simulink model "q_heli_2d_open_loop"  (Simulink 7.7)
settings: Solver=ode1  StartTime=0.0  StopTime=inf  FixedStep=0.002  RelTol=1e-3
values from neighbouring files (symbols this model uses):
  JOYSTICK_X_DZ = 0.25    [setup_lab_heli_2d.m]
  JOYSTICK_Y_DZ = 0.25    [setup_lab_heli_2d.m]
  K_AMP = 3    [setup_lab_heli_2d.m]
  K_EC_P = - 2 * pi / ( 4 * 1024 )    (= -0.00153398078789)    [setup_lab_heli_2d.m]
  K_EC_Y = 2 * pi / ( 8 * 1024 )    (= 0.000766990393943)    [setup_lab_heli_2d.m]
  K_JOYSTICK_V_X = 10    [setup_lab_heli_2d.m]
  K_JOYSTICK_V_Y = 5    [setup_lab_heli_2d.m]
  theta_0 = -40.5*pi/180    (= -0.706858347058)    [setup_lab_heli_2d.m]
  VMAX_AMP_P = 24    [setup_lab_heli_2d.m]
  VMAX_AMP_Y = 15    [setup_lab_heli_2d.m]
  wcf = 2 * pi * 20    (= 125.663706144)    [setup_lab_heli_2d.m]
  zetaf = 0.85    [setup_lab_heli_2d.m]
undefined symbols (not defined in the file or in its folder): HIL, qc_get_step_size
libraries: quarc_library x4, simulink_extras x3
settings Model: Creator=MLevis  LastModifiedBy=pmartin  SimulationMode=external  ExtModeTrigDuration=50000  BufferReuse=off
settings SolverCC: PositivePriorityOrder=on
settings OptimizationCC: BooleanDataType=off  InlineInvariantSignals=on  OptimizeBlockIOStorage=off  BufferReuse=off  ExpressionFolding=off  LocalBlockOutputs=off  InitFltsAndDblsToZero=on
settings DebuggingCC: SaveWithParameterizedLinksMsg=none  SignalResolutionControl=TryResolveAllWithWarning  MultiTaskDSMMsg=warning  MultiTaskCondExecSysMsg=none  StrictBusMsg=None
settings RTWCC: SystemTargetFile=quarc_windows.tlc  TemplateMakefile=quarc_default_tmf  Description=QuaRC Win32 Target  ProcessScript=quarc_windows_make_rtw_hook  IncludeERTFirstTime=on
settings STFCustomTargetCC: TargetFcnLib=ansi_tfl_tmw.mat  TargetPreCompLibLocation=C:\PROGRA~3\QUARC\lib\2012b\windows\release  GeneratePreprocessorConditionals=Disable all  SystemTargetFile=quarc_windows.tlc
settings GRTTargetCC: TargetFcnLib=ansi_tfl_tmw.mat  TargetPreCompLibLocation=C:\PROGRA~3\QUARC\lib\2012b\windows\release  ParMdlRefBuildCompliant=off  CompOptLevelCompliant=off  MatFileLogging=off  ExtMode=on  ExtModeMexFile=quarc_comm

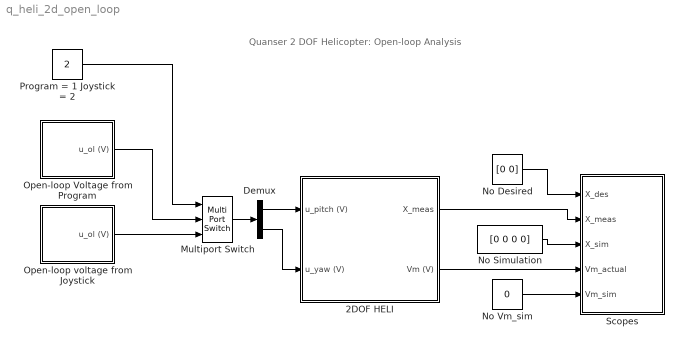
== system q_heli_2d_open_loop ==
  note: Quanser 2 DOF Helicopter:
      | Open-loop Analysis
  2DOF HELI : Subsystem
  Demux : Demux  Outputs=2
  Multiport Switch : MultiPortSwitch  Inputs=2
  No Desired : Constant  Value=[0 0]
  No Simulation : Constant  Value=[0 0 0 0]
  No Vm_sim : Constant  Value=0
  Open-loop Voltage from Program : Subsystem
  Open-loop voltage from Joystick : Subsystem
  Program = 1 Joystick = 2 : Constant  Value=2
  Scopes : Subsystem
  wires:
  Open-loop Voltage from Program/1(u_ol (V)) -> Multiport Switch/2
  Program = 1 Joystick = 2/1 -> Multiport Switch/1
  Open-loop voltage from Joystick/1(u_ol (V)) -> Multiport Switch/3
  Multiport Switch/1 -> Demux/1
  Demux/1 -> 2DOF HELI/1(u_pitch (V))
  Demux/2 -> 2DOF HELI/2(u_yaw (V))
  2DOF HELI/1(X_meas) -> Scopes/2(X_meas)
  2DOF HELI/2(Vm (V)) -> Scopes/4(Vm_actual)
  No Desired/1 -> Scopes/1(X_des)
  No Simulation/1 -> Scopes/3(X_sim)
  No Vm_sim/1 -> Scopes/5(Vm_sim)

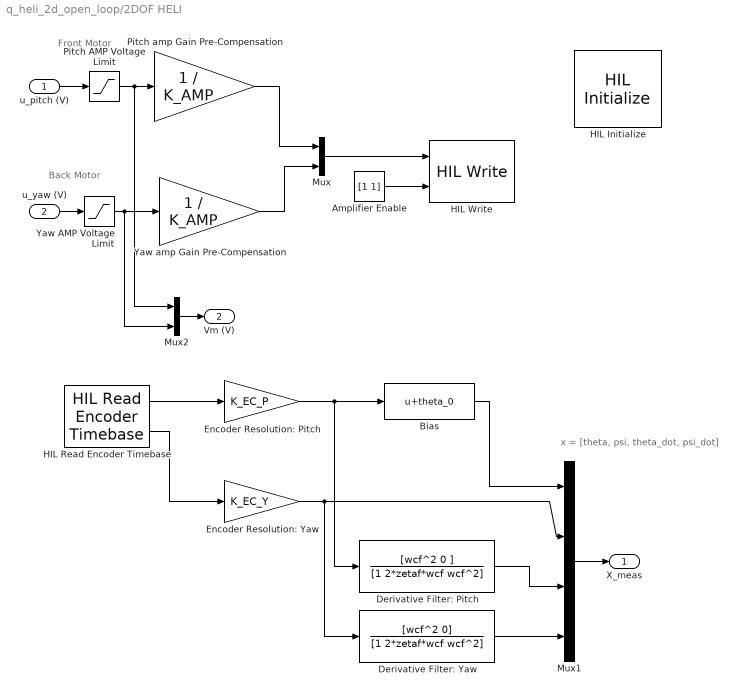
== system q_heli_2d_open_loop/2DOF HELI ==
  note: Back Motor
  note: Front Motor
  note: x = [theta, psi, theta_dot, psi_dot]
  u_pitch (V) : Inport
  u_yaw (V) : Inport  Port=2
  Amplifier Enable : Constant  Value=[1 1]
  Bias : Bias  Bias=theta_0
  Derivative Filter: Pitch : TransferFcn  Numerator=[wcf^2 0 ]  Denominator=[1 2*zetaf*wcf wcf^2]
  Derivative Filter: Yaw : TransferFcn  Numerator=[wcf^2 0]  Denominator=[1 2*zetaf*wcf wcf^2]
  "Encoder Resolution: Pitch " : Gain  Gain=K_EC_P
  Encoder Resolution: Yaw : Gain  Gain=K_EC_Y
  HIL Initialize : quarc_library/Data Acquisition/Generic/Configuration/HIL Initialize  object_name=HIL-1  board_type=q2_usb  board_number=0  board_options=d0=digital;d1=digital;led=auto;update_rate=normal;decimation=1  exclusive=off  active=on  hardware_clocks=[0]  clock_modes=[]  initial_clock_frequencies=[]  set_clock_params_at_start=off  set_clock_params_at_switch_in=off  set_clock_frequencies_at_start=off  set_clock_frequencies_at_switch_in=off  analog_input_channels=[0:1]  analog_input_maximums=10  analog_input_minimums=-10  set_analog_input_params_at_start=on  set_analog_input_params_at_switch_in=off  analog_output_channels=[0:1]  analog_output_maximums=10  analog_output_minimums=-10  initial_analog_outputs=[0]  final_analog_outputs=[0]  watchdog_analog_outputs=0  set_analog_output_params_at_start=on  set_analog_output_params_at_switch_in=off  set_analog_outputs_at_start=on  set_analog_outputs_at_switch_in=off  set_analog_outputs_at_terminate=on  set_analog_outputs_at_switch_out=off  set_analog_outputs_on_watchdog=off  digital_input_channels=[]  digital_output_channels=[0:1]  digital_output_configuration=[]  initial_digital_outputs=[0]  final_digital_outputs=[0]  watchdog_digital_outputs=[0]  set_digital_output_params_at_start=off  set_digital_output_params_at_switch_in=off  set_digital_outputs_at_start=on  set_digital_outputs_at_switch_in=off  set_digital_outputs_at_terminate=on  set_digital_outputs_at_switch_out=off  set_digital_outputs_on_watchdog=on  encoder_channels=[0:1]  quadrature=[4]  encoder_filter_frequency=[]  initial_encoder_counts=[0]  set_encoder_params_at_start=on  set_encoder_params_at_switch_in=off  set_encoder_counts_at_start=on  set_encoder_counts_at_switch_in=off  pwm_channels=[]  pwm_modes=[0]  pwm_frequency=1/0.020  pwm_configuration=[]  pwm_alignment=[]  pwm_polarity=[]  pwm_leading_deadband=[]  pwm_trailing_deadband=[]  initial_pwm_outputs=[0]  final_pwm_outputs=[0]  watchdog_pwm_outputs=[0]  set_pwm_params_at_start=on  set_pwm_params_at_switch_in=off  set_pwm_outputs_at_start=on  set_pwm_outputs_at_switch_in=off  set_pwm_outputs_at_terminate=on  set_pwm_outputs_at_switch_out=off  set_pwm_outputs_on_watchdog=off  other_output_channels=[]  initial_other_outputs=[]  final_other_outputs=[]  watchdog_other_outputs=[]  set_other_outputs_at_start=off  set_other_outputs_at_switch_in=off  set_other_outputs_at_terminate=off  set_other_outputs_at_switch_out=off  set_other_outputs_on_watchdog=off
  HIL Read Encoder Timebase : quarc_library/Data Acquisition/Generic/Timebases/HIL Read Encoder Timebase  object_name=HIL-1  clock=0  channels=[0:1]  samples_in_buffer=max(ceil(1/qc_get_step_size), 1)  active=on  vector_output=off  data_type_mode=Inherit via back propagation  data_type=double
  HIL Write : quarc_library/Data Acquisition/Generic/Immediate I//O/HIL Write  object_name=HIL-1  analog_channels=[0:1]  pwm_channels=[]  digital_channels=[0:1]  other_channels=[]  sample_time=-1  active=off  vector_input=on
  Mux : Mux  Inputs=2
  Mux1 : Mux
  Mux2 : Mux  Inputs=2
  Pitch AMP Voltage Limit : Saturate  UpperLimit=VMAX_AMP_P  LowerLimit=- VMAX_AMP_P
  Pitch amp Gain Pre-Compensation : Gain  Gain=1 / K_AMP  SaturateOnIntegerOverflow=on  OutDataTypeStr=Inherit: Same as input  ParamDataTypeStr=Inherit: Same as input
  Yaw AMP Voltage Limit : Saturate  UpperLimit=VMAX_AMP_Y  LowerLimit=- VMAX_AMP_Y
  Yaw amp Gain Pre-Compensation : Gain  Gain=1 / K_AMP  SaturateOnIntegerOverflow=on  OutDataTypeStr=Inherit: Same as input  ParamDataTypeStr=Inherit: Same as input
  X_meas : Outport
  Vm (V) : Outport  Port=2
  wires:
  Amplifier Enable/1 -> HIL Write/2
  Encoder Resolution: Yaw/1 -> Mux1/2, Derivative Filter: Yaw/1
  Mux2/1 -> Vm (V)/1
  Yaw amp Gain Pre-Compensation/1 -> Mux/2
  Pitch amp Gain Pre-Compensation/1 -> Mux/1
  Mux1/1 -> X_meas/1
  u_yaw (V)/1 -> Yaw AMP Voltage Limit/1
  u_pitch (V)/1 -> Pitch AMP Voltage Limit/1
  Yaw AMP Voltage Limit/1 -> Mux2/2, Yaw amp Gain Pre-Compensation/1
  Pitch AMP Voltage Limit/1 -> Mux2/1, Pitch amp Gain Pre-Compensation/1
  Mux/1 -> HIL Write/1
  HIL Read Encoder Timebase/1 -> "Encoder Resolution: Pitch "/1
  "Encoder Resolution: Pitch "/1 -> Bias/1, Derivative Filter: Pitch/1
  HIL Read Encoder Timebase/2 -> Encoder Resolution: Yaw/1
  Bias/1 -> Mux1/1
  Derivative Filter: Pitch/1 -> Mux1/3
  Derivative Filter: Yaw/1 -> Mux1/4

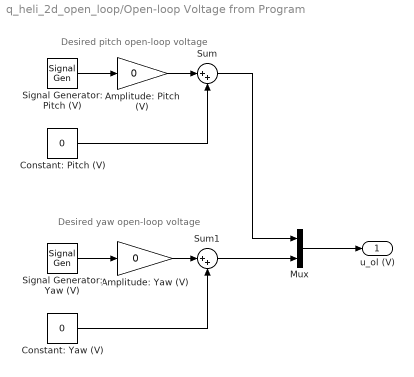
== system q_heli_2d_open_loop/Open-loop Voltage from Program ==
  note: Desired yaw open-loop voltage
  note: Desired pitch open-loop voltage
  Amplitude: Pitch (V) : Gain  Gain=0
  Amplitude: Yaw (V) : Gain  Gain=0
  Constant: Pitch (V) : Constant  Value=0
  Constant: Yaw (V) : Constant  Value=0
  Mux : Mux  Inputs=2
  Signal Generator: Pitch (V) : SignalGenerator  WaveForm=square  Frequency=0.4
  Signal Generator: Yaw (V) : SignalGenerator  WaveForm=square  Frequency=0.01
  Sum : Sum  Inputs=|++
  Sum1 : Sum  Inputs=|++
  u_ol (V) : Outport
  wires:
  Mux/1 -> u_ol (V)/1
  Sum1/1 -> Mux/2
  Sum/1 -> Mux/1
  Signal Generator: Yaw (V)/1 -> Amplitude: Yaw (V)/1
  Amplitude: Yaw (V)/1 -> Sum1/1
  Constant: Yaw (V)/1 -> Sum1/2
  Signal Generator: Pitch (V)/1 -> Amplitude: Pitch (V)/1
  Amplitude: Pitch (V)/1 -> Sum/1
  Constant: Pitch (V)/1 -> Sum/2

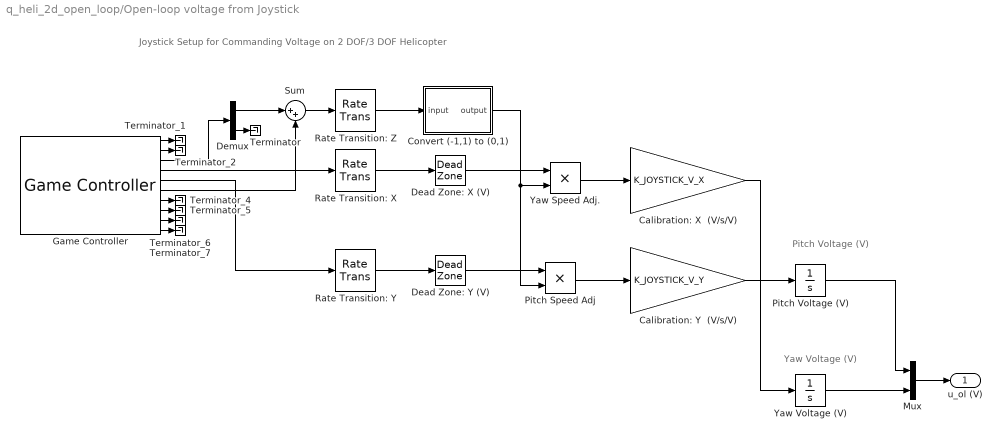
== system q_heli_2d_open_loop/Open-loop voltage from Joystick ==
  note: Joystick Setup for Commanding Voltage on 2 DOF/3 DOF Helicopter
  note: Yaw Voltage (V)
  note: Pitch Voltage (V)
  Calibration: X  (V/s/V) : Gain  Gain=K_JOYSTICK_V_X
  Calibration: Y  (V/s/V) : Gain  Gain=K_JOYSTICK_V_Y
  Convert (-1,1) to (0,1) : Subsystem
  Dead Zone: X (V) : DeadZone  LowerValue=-JOYSTICK_X_DZ  UpperValue=JOYSTICK_X_DZ  SaturateOnIntegerOverflow=on
  Dead Zone: Y (V) : DeadZone  LowerValue=-JOYSTICK_Y_DZ  UpperValue=JOYSTICK_Y_DZ  SaturateOnIntegerOverflow=on
  Demux : Demux  Outputs=2
  Game Controller : quarc_library/Devices/Peripherals/Target/Game Controller  controller=1  buffer_size=12  deadzone=[]  saturation=[]  sample_time=max(qc_get_step_size, 0.01)  auto_center=off  enabled=on
  Mux : Mux  Inputs=2
  Pitch Speed Adj : Product  RndMeth=Zero
  Pitch Voltage (V) : Integrator  LimitOutput=on  UpperSaturationLimit=VMAX_AMP_P  LowerSaturationLimit=-VMAX_AMP_P
  Rate Transition: X : RateTransition
  Rate Transition: Y : RateTransition
  Rate Transition: Z : RateTransition
  Sum : Sum  Inputs=|++
  Terminator : Terminator
  Terminator_{1..2,4..7} (6 alike) : Terminator
  Yaw Speed Adj. : Product  RndMeth=Zero
  Yaw Voltage (V) : Integrator  LimitOutput=on  UpperSaturationLimit=VMAX_AMP_Y  LowerSaturationLimit=-VMAX_AMP_Y
  u_ol (V) : Outport
  wires:
  Convert (-1,1) to (0,1)/1(output) -> Pitch Speed Adj/2, Yaw Speed Adj./2
  Calibration: Y  (V/s/V)/1 -> Pitch Voltage (V)/1
  Pitch Speed Adj/1 -> Calibration: Y  (V/s/V)/1
  Yaw Speed Adj./1 -> Calibration: X  (V/s/V)/1
  Dead Zone: Y (V)/1 -> Pitch Speed Adj/1
  Dead Zone: X (V)/1 -> Yaw Speed Adj./1
  Calibration: X  (V/s/V)/1 -> Yaw Voltage (V)/1
  Pitch Voltage (V)/1 -> Mux/1
  Yaw Voltage (V)/1 -> Mux/2
  Mux/1 -> u_ol (V)/1
  Rate Transition: Z/1 -> Convert (-1,1) to (0,1)/1(input)
  Rate Transition: X/1 -> Dead Zone: X (V)/1
  Rate Transition: Y/1 -> Dead Zone: Y (V)/1
  Game Controller/5 -> Rate Transition: Y/1
  Game Controller/4 -> Rate Transition: X/1
  Game Controller/1 -> Terminator_1/1
  Game Controller/2 -> Terminator_2/1
  Game Controller/7 -> Terminator_4/1
  Game Controller/8 -> Terminator_5/1
  Game Controller/9 -> Terminator_6/1
  Game Controller/10 -> Terminator_7/1
  Sum/1 -> Rate Transition: Z/1
  Game Controller/6 -> Sum/2
  Demux/1 -> Sum/1
  Game Controller/3 -> Demux/1
  Demux/2 -> Terminator/1

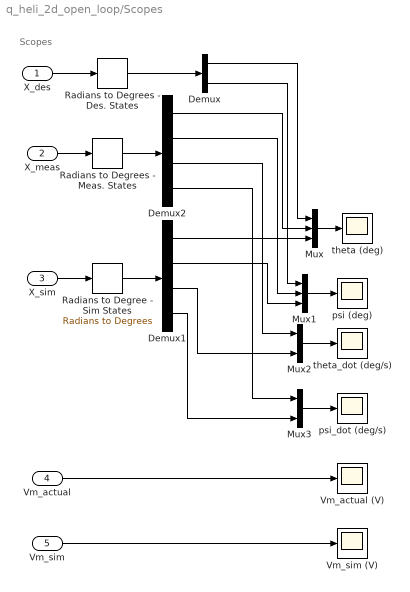
== system q_heli_2d_open_loop/Scopes ==
  note: Scopes
  X_des : Inport
  X_meas : Inport  Port=2
  X_sim : Inport  Port=3
  Vm_actual : Inport  Port=4
  Vm_sim : Inport  Port=5
  Demux : Demux  Outputs=2
  Demux1 : Demux
  Demux2 : Demux
  Mux : Mux  Inputs=3
  Mux1 : Mux  Inputs=3
  Mux2 : Mux  Inputs=2
  Mux3 : Mux  Inputs=2
  Radians to Degree - Sim States : simulink_extras/Transformations/Radians to Degrees
  Radians to Degrees - Des. States : simulink_extras/Transformations/Radians to Degrees
  Radians to Degrees - Meas. States : simulink_extras/Transformations/Radians to Degrees
  Vm_actual (V) : Scope
      settings: TickLabels=on  TimeRange=1.000000  YMin=-250  YMax=250  SaveName=ScopeData4
  Vm_sim (V) : Scope
      settings: TickLabels=on  TimeRange=1.000000  YMin=-250  YMax=250  SaveName=ScopeData5
  psi (deg) : Scope
      settings: TickLabels=on  TimeRange=50  YMin=-5.5  YMax=5.5
  psi_dot (deg/s) : Scope
      settings: TickLabels=on  TimeRange=1.000000  YMin=-250  YMax=250  SaveName=ScopeData3
  theta (deg) : Scope
      settings: TickLabels=on  TimeRange=50  YMin=-15  YMax=15
  theta_dot (deg/s) : Scope
      settings: TickLabels=on  TimeRange=1.000000  YMin=-250  YMax=250  SaveName=ScopeData2
  wires:
  Vm_sim/1 -> Vm_sim (V)/1
  Radians to Degrees - Des. States/1 -> Demux/1
  Demux1/2 -> Mux1/3
  Demux2/2 -> Mux1/2
  Demux/2 -> Mux1/1
  Demux1/1 -> Mux/3
  Demux2/1 -> Mux/2
  Demux/1 -> Mux/1
  X_des/1 -> Radians to Degrees - Des. States/1
  Demux2/3 -> Mux2/1
  Demux2/4 -> Mux3/1
  X_meas/1 -> Radians to Degrees - Meas. States/1
  Radians to Degrees - Meas. States/1 -> Demux2/1
  X_sim/1 -> Radians to Degree - Sim States/1
  Radians to Degree - Sim States/1 -> Demux1/1
  Mux/1 -> theta (deg)/1
  Mux1/1 -> psi (deg)/1
  Mux2/1 -> theta_dot (deg/s)/1
  Mux3/1 -> psi_dot (deg/s)/1
  Demux1/3 -> Mux2/2
  Demux1/4 -> Mux3/2
  Vm_actual/1 -> Vm_actual (V)/1

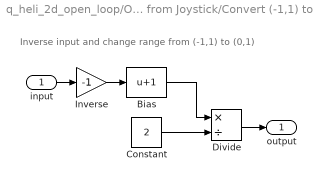
== system q_heli_2d_open_loop/Open-loop voltage from Joystick/Convert (-1,1) to (0,1) ==
  note: Inverse input and change range from (-1,1) to (0,1)
  input : Inport
  Bias : Bias  Bias=1
  Constant : Constant  Value=2
  Divide : Product  Inputs=*/
  Inverse : Gain  Gain=-1
  output : Outport
  wires:
  Inverse/1 -> Bias/1
  Divide/1 -> output/1
  input/1 -> Inverse/1
  Bias/1 -> Divide/1
  Constant/1 -> Divide/2
